simulink model "Main_circuit"  (R2025a)
settings: Solver=VariableStepAuto  StartTime=0.0  StopTime=60e-5  RelTol=1e-3
libraries: spsCurrentMeasurementLib x11, spsVoltageMeasurementLib x9, spsSeriesRLCBranchLib x4, spsDiodeLib x3, spsMosfetLib x3, spsDCVoltageSourceLib x1, spsLinearTransformerLib x1, spspowerguiLib x1
settings Model: LastModifiedBy=mithu

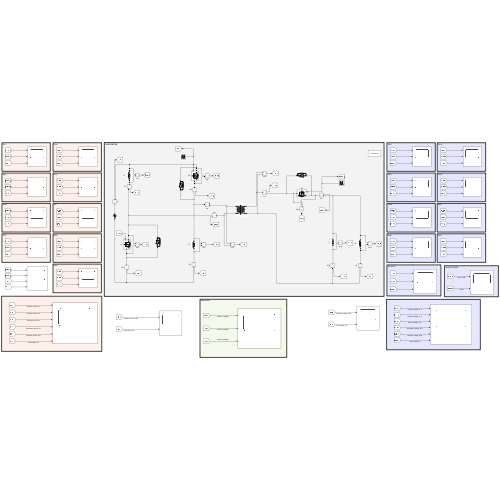
[thumbnail: Simulink's stored preview of the top-level diagram]
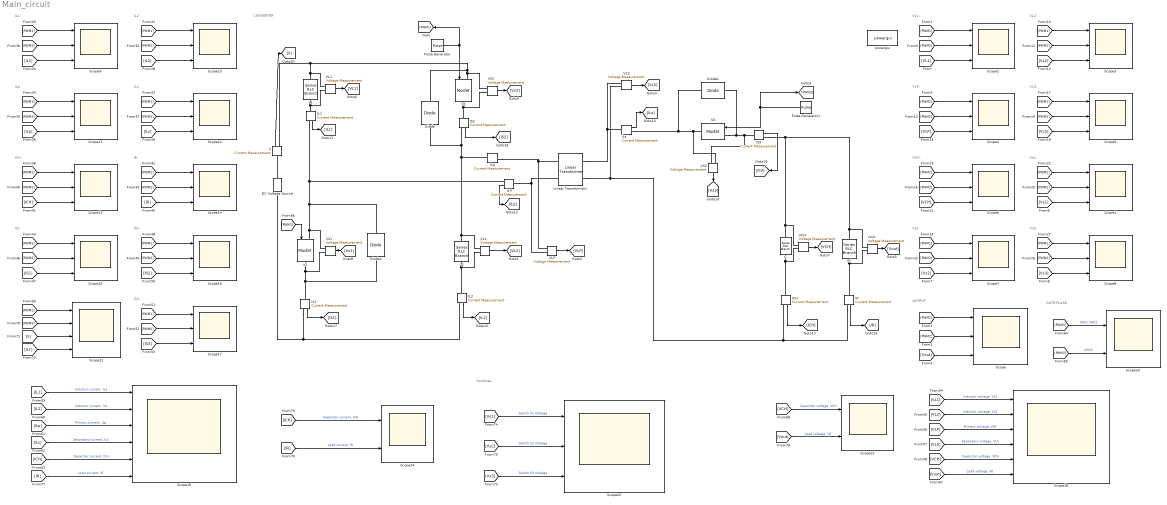
== system Main_circuit ==
  note: CONVERTER
  note: OUTPUT
  note: VL1:
  note: VL2:
  note: VLP:
  note: VLS:
  note: VCH:
  note: Vs1:
  note: Vs2:
  note: Vs3:
  note: IL1:
  note: IL2:
  note: ILp:
  note: ILs:
  note: ICH:
  note: IR:
  note: IS1:
  note: IS2:
  note: IS3:
  note: GATE PULSE:
  note: Switches:
  C : spsSeriesRLCBranchLib/Series RLC Branch  LConnTagsString=__new0  RConnTagsString=__new0  BranchType=C  Resistance=1  Inductance=1e-3  SetiL0=off  InitialCurrent=0  Capacitance=150e-6  Setx0=on  InitialVoltage=48  Measurements=Branch voltage and current
  DC Voltage Source : spsDCVoltageSourceLib/DC Voltage Source  Amplitude=12  Measurements=Voltage
  Diode : spsDiodeLib/Diode  Ron=0.001  Lon=0  Vf=1.2  IC=0  UseSnubber=0  Rs=2  Cs=10e-6  Measurements=off
  Diode1 : spsDiodeLib/Diode  Ron=0.001  Lon=0  Vf=1.2  IC=0  UseSnubber=0  Rs=2  Cs=10e-6  Measurements=off
  Diode2 : spsDiodeLib/Diode  Ron=0.001  Lon=0  Vf=0.8  IC=0  UseSnubber=0  Rs=2  Cs=10e-6  Measurements=off
  ICH : spsCurrentMeasurementLib/Current Measurement  PhasorSimulation=off  OutputType=Complex  PSBequivalent=0
  IL1 : spsCurrentMeasurementLib/Current Measurement  PhasorSimulation=off  OutputType=Complex  PSBequivalent=0
  IL2 : spsCurrentMeasurementLib/Current Measurement  PhasorSimulation=off  OutputType=Complex  PSBequivalent=0
  IL4 : spsCurrentMeasurementLib/Current Measurement  PhasorSimulation=off  OutputType=Complex  PSBequivalent=0
  ILp : spsCurrentMeasurementLib/Current Measurement  PhasorSimulation=off  OutputType=Complex  PSBequivalent=0
  IR : spsCurrentMeasurementLib/Current Measurement  PhasorSimulation=off  OutputType=Complex  PSBequivalent=0
  IS1 : spsCurrentMeasurementLib/Current Measurement  PhasorSimulation=off  OutputType=Complex  PSBequivalent=0
  IS2 : spsCurrentMeasurementLib/Current Measurement  PhasorSimulation=off  OutputType=Complex  PSBequivalent=0
  IS3 : spsCurrentMeasurementLib/Current Measurement  PhasorSimulation=off  OutputType=Complex  PSBequivalent=0
  Ii : spsCurrentMeasurementLib/Current Measurement  PhasorSimulation=off  OutputType=Complex  PSBequivalent=0
  L1 : spsSeriesRLCBranchLib/Series RLC Branch  LConnTagsString=__new0  RConnTagsString=__new0  BranchType=L  Resistance=1  Inductance=144e-6  SetiL0=off  InitialCurrent=16.67  Capacitance=1e-6  Setx0=off  InitialVoltage=0  Measurements=Branch voltage and current
  L2 : spsSeriesRLCBranchLib/Series RLC Branch  LConnTagsString=__new0  RConnTagsString=__new0  BranchType=L  Resistance=1  Inductance=144e-6  SetiL0=off  InitialCurrent=16.67  Capacitance=1e-6  Setx0=off  InitialVoltage=0  Measurements=None
  Linear Transformer1 : spsLinearTransformerLib/Linear Transformer  UNITS=SI  NominalPower=[ 100 50000 ]  winding1=[12 0.1 288e-6 ]  winding2=[48 0.1 4.608e-3]  ThreeWindings=off  winding3=[3.15e+05 0.7938 0.084225]  RmLm=[ 10e6 10e6]  Measurements=None  DataType=on
  Pulse Generator : DiscretePulseGenerator  PulseType=Time based  Period=20e-6  PulseWidth=50
  Pulse Generator1 : DiscretePulseGenerator  PulseType=Time based  Period=20e-6  PulseWidth=50  PhaseDelay=10e-6
  Rl : spsSeriesRLCBranchLib/Series RLC Branch  LConnTagsString=__new0  RConnTagsString=__new0  BranchType=R  Resistance=12  Inductance=1e-3  SetiL0=off  InitialCurrent=0  Capacitance=1e-6  Setx0=off  InitialVoltage=0  Measurements=None
  S2 : spsMosfetLib/Mosfet  Ron=11e-3  Lon=0  Rd=2.2e-3  Vfd=1.2  IC=0  Rs=1e4  Cs=inf  Measurements=off
  S3 : spsMosfetLib/Mosfet  Ron=11e-3  Lon=0  Rd=2.2e-3  Vfd=1.2  IC=0  Rs=1e5  Cs=inf  Measurements=off
  Scope{,1..17,22} (19 alike) : Scope  NumInputPorts=3
      Scope settings: ActiveDisplayYMinimum=-0.12499999999999997  ActiveDisplayYMaximum=1.125
      Scope1 settings: ActiveDisplayString=3  ActiveDisplayYMinimum=-5.0879947508123431  ActiveDisplayYMaximum=47.205399003366871
      Scope10 settings: ActiveDisplayString=3  ActiveDisplayYMinimum=-0.80965427488447816  ActiveDisplayYMaximum=7.3181276630605634  DataLoggingVariableName=ScopeData10
      Scope11 settings: ActiveDisplayString=3  ActiveDisplayYMinimum=-123.51802810916602  ActiveDisplayYMaximum=-119.52868385951439  DataLoggingVariableName=ScopeData11
      Scope12 settings: ActiveDisplayString=3  ActiveDisplayYMinimum=-0.42447919821768282  ActiveDisplayYMaximum=0.050111586738149479  DataLoggingVariableName=ScopeData12
      Scope13 settings: ActiveDisplayString=3  ActiveDisplayYMinimum=-2.3759587865393441  ActiveDisplayYMaximum=-1.9181702032339496  DataLoggingVariableName=ScopeData13
      Scope14 settings: ActiveDisplayString=3  ActiveDisplayYMinimum=1.9368881178808768  ActiveDisplayYMaximum=2.0996050239391613  DataLoggingVariableName=ScopeData14
      Scope15 settings: ActiveDisplayString=3  ActiveDisplayYMinimum=-6.048955858619725  ActiveDisplayYMaximum=54.45260272748984  DataLoggingVariableName=ScopeData15
      Scope16 settings: ActiveDisplayString=3  ActiveDisplayYMinimum=-24.934746809239325  ActiveDisplayYMaximum=224.41297385608692  DataLoggingVariableName=ScopeData16
      Scope17 settings: ActiveDisplayString=3  ActiveDisplayYMinimum=-1.2684458715440969  ActiveDisplayYMaximum=11.382581351659036  DataLoggingVariableName=ScopeData17
      Scope2 settings: ActiveDisplayString=3  ActiveDisplayYMinimum=-2.541300043116228  ActiveDisplayYMaximum=13.461717595271965  DataLoggingVariableName=ScopeData2
      Scope22 settings: ActiveDisplayYMinimum=-1.6537237540128014  ActiveDisplayYMaximum=14.968660165282738  DataLoggingVariableName=ScopeData22
      Scope3 settings: ActiveDisplayString=3  ActiveDisplayYMinimum=-2.5900016821164842  ActiveDisplayYMaximum=14.954444631331938  DataLoggingVariableName=ScopeData3
      Scope4 settings: ActiveDisplayString=3  ActiveDisplayYMinimum=-37.05882597636711  ActiveDisplayYMaximum=17.432069801203717  DataLoggingVariableName=ScopeData4
      Scope5 settings: ActiveDisplayString=3  ActiveDisplayYMinimum=38.024698152327019  ActiveDisplayYMaximum=49.731010573967055  DataLoggingVariableName=ScopeData5
      Scope6 settings: ActiveDisplayString=3  ActiveDisplayYMinimum=44.6259022359754  ActiveDisplayYMaximum=48.374899751558289  DataLoggingVariableName=ScopeData6
      Scope7 settings: ActiveDisplayString=3  ActiveDisplayYMinimum=-5.08799475070775  ActiveDisplayYMaximum=47.205399002425523  DataLoggingVariableName=ScopeData7
      Scope8 settings: ActiveDisplayString=3  ActiveDisplayYMinimum=-0.90066873295261085  ActiveDisplayYMaximum=0.10005694283632297  DataLoggingVariableName=ScopeData8
      Scope9 settings: ActiveDisplayString=3  ActiveDisplayYMinimum=-5.7970599321119556  ActiveDisplayYMaximum=52.204779708575053  DataLoggingVariableName=ScopeData9
  Scope18 : Scope  NumInputPorts=6
      settings: ActiveDisplayString=6  ActiveDisplayYMinimum=28.241763066261  ActiveDisplayYMaximum=50.195359659304337  DataLoggingVariableName=ScopeData18
  Scope19 : Scope  NumInputPorts=6
      settings: ActiveDisplayString=6  ActiveDisplayYMinimum=3.2478710268851634  ActiveDisplayYMaximum=4.0835698859016487  DataLoggingVariableName=ScopeData19
  Scope20 : Scope  NumInputPorts=2
      settings: ActiveDisplayYMinimum=-0.12499999999999997  ActiveDisplayYMaximum=1.125  DataLoggingVariableName=ScopeData20
  Scope21 : Scope  NumInputPorts=4
      settings: ActiveDisplayString=3  ActiveDisplayYMinimum=-171.1279899457345  ActiveDisplayYMaximum=1519.1734223679923  DataLoggingVariableName=ScopeData21
  Scope23 : Scope  NumInputPorts=2
      settings: ActiveDisplayYMinimum=47.163892623622075  ActiveDisplayYMaximum=53.6273765764084  DataLoggingVariableName=ScopeData23
  Scope24 : Scope  NumInputPorts=2
      settings: ActiveDisplayYMinimum=-3.1254799181046664  ActiveDisplayYMaximum=5.6703992460350232  DataLoggingVariableName=ScopeData24
  VCH : spsVoltageMeasurementLib/Voltage Measurement  PhasorSimulation=off  OutputType=Complex  PSBequivalent=0
  VL1 : spsVoltageMeasurementLib/Voltage Measurement  PhasorSimulation=off  OutputType=Complex  PSBequivalent=0
  VL2 : spsVoltageMeasurementLib/Voltage Measurement  PhasorSimulation=off  OutputType=Complex  PSBequivalent=0
  VLP : spsVoltageMeasurementLib/Voltage Measurement  PhasorSimulation=off  OutputType=Complex  PSBequivalent=0
  VLS : spsVoltageMeasurementLib/Voltage Measurement  PhasorSimulation=off  OutputType=Complex  PSBequivalent=0
  VS1 : spsVoltageMeasurementLib/Voltage Measurement  PhasorSimulation=off  OutputType=Complex  PSBequivalent=0
  VS2 : spsVoltageMeasurementLib/Voltage Measurement  PhasorSimulation=off  OutputType=Complex  PSBequivalent=0
  VS3 : spsVoltageMeasurementLib/Voltage Measurement  PhasorSimulation=off  OutputType=Complex  PSBequivalent=0
  Vout : spsVoltageMeasurementLib/Voltage Measurement  PhasorSimulation=off  OutputType=Complex  PSBequivalent=0
  iLs : spsCurrentMeasurementLib/Current Measurement  PhasorSimulation=off  OutputType=Complex  PSBequivalent=0
  powergui : spspowerguiLib/powergui  Priority=1  SimulationMode=Continuous  SampleTime=50e-6  frequency=60  Iterations=50  frequencyindice=0  Pbase=100e6  ErrMax=1e-4  UnitsV=kV  UnitsW=MW  buscounter=0  FunctionMessages=off  echomessages=off  EnableUseOfTLC=off  CurrentSourceSwitches=off  DisableSnubberDevices=off  DisableRonSwitches=off  DisableVfSwitches=off  DisplayEquations=off  AutomaticDiscreteSolvers=off  SolverType=Tustin/Backward Euler (TBE)  Interpol=off  ExternalGateDelay=off  methode=off  Ts=100  x0status=blocks  SPID=on  SwTol=0  HookPort=off  NonlinearTolerance=1e-4  nMaxIteration=100  ContinueOnMaxIteration=off  RestoreLinks=warning  ResistiveCurrentMeasurement=off  Frange=[0:2:500]  Ylog=off  Xlog=on  ShowGrid=off  save=off  variable=ZData  structure=0  ZoomFFT=off  StartTime=0.0  cycles=1  DisplayStyle=1  fundamental=60  FreqAxis=off  MaxFrequency=1000  frequencyindicesteady=1  RmsSteady=1  display=off
  s1 : spsMosfetLib/Mosfet  Ron=11e-3  Lon=0  Rd=2.2e-3  Vfd=1.2  IC=0  Rs=1e4  Cs=inf  Measurements=off
  wires:
  Vout/1 -> [Vout]
  Pulse Generator1/1 -> [PWM2], S3/1
  [PWM1] -> Scope/1
  [PWM2] -> Scope/2
  [Vout] -> Scope/3
  Pulse Generator/1 -> S2/1, [PWM1]
  [VL1] -> Scope2/3
  [PWM1] -> Scope2/1
  [PWM2] -> Scope2/2
  VL1/1 -> [VL1]
  [PWM2] -> Scope3/2
  [PWM1] -> Scope3/1
  [VL2] -> Scope3/3
  VL2/1 -> [VL2]
  [VLP] -> Scope4/3
  [PWM1] -> Scope4/1
  [PWM2] -> Scope4/2
  VLP/1 -> [VLP]
  VLS/1 -> [VLS]
  [PWM2] -> Scope5/2
  [PWM1] -> Scope5/1
  [VLS] -> Scope5/3
  [VCH] -> Scope6/3
  [PWM1] -> Scope6/1
  [PWM2] -> Scope6/2
  VCH/1 -> [VCH]
  VS1/1 -> [Vs1]
  VS2/1 -> [Vs2]
  VS3/1 -> [Vs3]
  [PWM2] -> Scope1/2
  [PWM1] -> Scope1/1
  [Vs1] -> Scope1/3
  [Vs2] -> Scope7/3
  [PWM1] -> Scope7/1
  [PWM2] -> Scope7/2
  [PWM2] -> Scope8/2
  [PWM1] -> Scope8/1
  [Vs3] -> Scope8/3
  IL1/1 -> [IL1]
  [PWM2] -> Scope9/2
  [PWM1] -> Scope9/1
  [IL1] -> Scope9/3
  IL2/1 -> [IL2]
  [IL2] -> Scope10/3
  [PWM1] -> Scope10/1
  [PWM2] -> Scope10/2
  [PWM2] -> Scope11/2
  [PWM1] -> Scope11/1
  [ILp] -> Scope11/3
  [ILs] -> Scope12/3
  [PWM1] -> Scope12/1
  [PWM2] -> Scope12/2
  ICH/1 -> [ICH]
  IR/1 -> [IR]
  [PWM2] -> Scope13/2
  [PWM1] -> Scope13/1
  [ICH] -> Scope13/3
  [IR] -> Scope14/3
  [PWM1] -> Scope14/1
  [PWM2] -> Scope14/2
  [PWM2] -> Scope15/2
  [PWM1] -> Scope15/1
  [IS1] -> Scope15/3
  [IS2] -> Scope16/3
  [PWM1] -> Scope16/1
  [PWM2] -> Scope16/2
  [PWM2] -> Scope17/2
  [PWM1] -> Scope17/1
  [IS3] -> Scope17/3
  IS1/1 -> [IS1]
  IS2/1 -> [IS2]
  iLs/1 -> [ILs]
  IS3/1 -> [IS3]
  [VL1] -> Scope18/1  "Inductor voltage, VL1"
  [VL2] -> Scope18/2  "Inductor voltage, VL2"
  [VLP] -> Scope18/3  "Primary voltage, VLP"
  [VLS] -> Scope18/4  "Secondary voltage, VLS"
  [VCH] -> Scope18/5  "Capacitor voltage, VCH"
  [ICH] -> Scope19/5  "Capacitor current, ICH"
  [ILs] -> Scope19/4  "Secondary current, ILs"
  [ILp] -> Scope19/3  "Primary current, ILp"
  [IL2] -> Scope19/2  "Inductor current, IL2"
  [IL1] -> Scope19/1  "Inductor current, IL1"
  [PWM2] -> Scope20/2  "VGS3"
  [PWM1] -> Scope20/1  "VGS1,VGS2"
  Ii/1 -> [Ii]
  [Ii] -> Scope21/3
  [PWM1] -> Scope21/1
  [PWM2] -> Scope21/2
  [IL1] -> Scope21/4
  IL4/1 -> [ILp]
  [PWM1] -> s1/1
  [Vs3] -> Scope22/3  "Switch S3 Voltage"
  [Vs1] -> Scope22/1  "Switch S1 Voltage"
  [Vs2] -> Scope22/2  "Switch S2 Voltage"
  [Vout] -> Scope18/6  "Load voltage, V0"
  [IR] -> Scope19/6  "Load current, IR"
  [ICH] -> Scope24/1  "Capacitor current, ICH"
  [IR] -> Scope24/2  "Load current, IR"
  [VCH] -> Scope23/1  "Capacitor voltage, VCH"
  [Vout] -> Scope23/2  "Load voltage, V0"
  connections:
  C/LConn1 -- IS3/RConn1 -- Rl/LConn1 -- Vout/LConn1 -- VCH/LConn1
  iLs/RConn1 -- Diode2/RConn1 -- S3/RConn1 -- VS3/LConn1
  VL2/LConn2 -- IL2/LConn1 -- L2/RConn1
  VCH/LConn2 -- ICH/LConn1 -- C/RConn1
  IL1/LConn1 -- VL1/LConn2 -- L1/RConn1
  VS1/LConn2 -- s1/RConn1 -- Diode1/LConn1 -- IS1/LConn1
  L2/LConn1 -- Diode/LConn1 -- IS2/RConn1 -- ILp/LConn1 -- VL2/LConn1
  IL4/LConn1 -- VLP/LConn2 -- Linear Transformer1/LConn2
  IR/LConn1 -- Vout/LConn2 -- Rl/RConn1
  IS1/RConn1 -- DC Voltage Source/LConn1 -- IL2/RConn1
  VS2/LConn2 -- S2/RConn1 -- IS2/LConn1
  VS3/LConn2 -- Diode2/LConn1 -- S3/LConn1 -- IS3/LConn1
  L1/LConn1 -- VL1/LConn1 -- Ii/RConn1 -- Diode/RConn1 -- VS2/LConn1 -- S2/LConn1
  DC Voltage Source/RConn1 -- Ii/LConn1
  VS1/LConn1 -- Diode1/RConn1 -- IL1/RConn1 -- IL4/RConn1 -- s1/LConn1
  iLs/LConn1 -- Linear Transformer1/RConn1 -- VLS/LConn1
  Linear Transformer1/RConn2 -- VLS/LConn2 -- IR/RConn1 -- ICH/RConn1
  ILp/RConn1 -- VLP/LConn1 -- Linear Transformer1/LConn1
